simulink model "GHAME_Model_2018b"  (R2018b)
settings: Solver=ode2  StartTime=0.0  StopTime=Sim.simulation.duration  FixedStep=Sim.sample_time  RelTol=1e-3
undefined symbols (not defined in the file): Data, IC, Sim, UNC, v0_BE_B
libraries: simulink_extras x8, sharedutil x2
(part 2 of 2)

== matlab function GHAME_Model_2018b/GHAME Airframe/Forces and Moments/PROPULSION/Subsystem/Updating mass and inertia ==
  data: IBBB output size=[3 3]; IBBBdot output; fmdot input; fmasse input; vmass output size=[1 1]; Sim parameter; stop_flag output
function [IBBB, IBBBdot, vmass, stop_flag] = mass(fmdot, fmasse, Sim)
% mass
% -------------------------------------------------------------------------
% Updates the vehicle total mass, mass derivative, inertia tensor, and 
% inertia time derivative as a function of expended fuel. The mass 
% properties are interpolated between the full and empty tank conditions. 
% A stop flag is generated when the remaining fuel mass approaches zero.
%
% INPUTS:
%   fmdot   - Fuel mass flow rate (fuel consumption rate) [kg/s]
%   fmasse  - Expended fuel mass [kg]
%
% OUTPUTS:
%   vmass     - Current vehicle mass [kg]
%   vmassdot  - Time derivative of vehicle mass [kg/s]
%   IBBB      - Current inertia tensor [3x3]
%   IBBBdot   - Time derivative of inertia tensor [3x3/s]
%   stop_flag - Boolean flag (1 if fuel is exhausted, 0 otherwise)

fmass_init = Sim.vehicle.mass.fuel;
fmass_full = Sim.vehicle.mass.fuel_full;
vmass_init = Sim.vehicle.mass.current;
IBBB0  = Sim.vehicle.inertia.IBBB0;
IBBB1  = Sim.vehicle.inertia.IBBB1;

% Updating vehicle mass and fuel mass based on expended fuel
vmass = vmass_init - fmasse;       % Current vehicle mass
fmass = fmass_init - fmasse;       % Remaining fuel mass

% Time derivative of vehicle mass (negative fuel consumption rate)
vmassdot = -fmdot;

% Compute interpolation ratio (0 = full tank, 1 = empty tank)
mass_ratio = fmass / fmass_full;

% Difference in inertia between full and empty tank
dI = IBBB0 - IBBB1;

% Interpolate inertia tensor based on current fuel state
IBBB = IBBB1 + dI * mass_ratio;

% Compute inertia tensor time derivative using chain rule
IBBBdot = (-fmdot / fmass_full) * dI;

% Generate stop flag when fuel is nearly exhausted
stop_flag = (fmass <= 1e-6);

end

== matlab function GHAME_Model_2018b/GHAME Airframe/Environment/ENVIRONMENT/Wind and Turbulence/Wind Computation ==
  settings: updateMethod=CONTINUOUS
  data: Vwind input; VTAD input; VAEDS input; VAED output; Sim parameter; VAEDSD output
function [VAED, VAEDSD]  = wind(Vwind, VTAD, VAEDS, Sim)
    % Wind Computes atmospheric properties, wind, and turbulence.
    %
    % States:
    % VAED   - Wind velocity in geodetic coordinates - m/s
    % VAEDS  - Smoothed wind velocity in geodetic coord - m/s
    % VAEDSD - Smoothed wind velocity derivative - m/s

    mturb = Sim.mode.mturb;
    mwind = Sim.mode.mwind;
    
    % Constants
    twind = 10;           % Wind smoothing time constant
    if mwind > 0
        % Compute wind components in geodetic coordinates
        VAED_RAW = [Vwind(1);  % North (meridional)
                    Vwind(2);  % East  (zonal)
                    0];      % Vertical (positive up)
    
        % Smoothing wind by filtering with time constant 'twind' sec
        VAEDSD = (VAED_RAW - VAEDS) * (1 / twind);
        VAED   = VAEDS;
    else
        VAEDSD = [0; 0; 0];
        VAED   = [0; 0; 0];
    end
    
    % Add Dryden turbulence
    if mturb > 0
        VAED = VAED + VTAD;
    else 
    end

end

== matlab function GHAME_Model_2018b/GHAME Airframe/Environment/ENVIRONMENT/Gravity Calculation ==
  data: time input; SBII input; GRAVG output; IC parameter; Sim parameter
function GRAVG  = cad_grav84(time, SBII, IC, Sim)
  
    % Extract Constants
    SMAJOR_AXIS = Sim.earth.SMAJOR_AXIS;
    C20         = Sim.earth.C20;
    REARTH      = Sim.earth.REARTH;
    GW_CLONG    = Sim.earth.GW_CLONG;
    GM          = Sim.earth.GM;

    WEII3 = IC.WEII3;

    % Initialize output
    GRAVG = zeros(3,1);

    % Compute geocentric coordinates
    [lonc, latc, altc] = cad_geoc_in(SBII, time, REARTH, WEII3, GW_CLONG);

    % Compute the gravitational acceleration
    dbi = norm(SBII); % Magnitude of position vector
    dum1 = GM / (dbi^2);
    dum2 = 3 * sqrt(5);
    dum3 = (SMAJOR_AXIS / dbi)^2;

    gravg1 = -dum1 * dum2 * C20 * dum3 * sin(latc) * cos(latc);
    gravg2 = 0;
    gravg3 = dum1 * (1 + dum2 / 2 * C20 * dum3 * (3 * sin(latc)^2 - 1));

    % Assign values
    GRAVG(1) = gravg1;
    GRAVG(2) = gravg2;
    GRAVG(3) = gravg3;
end

function [lonc, latc, altc] = cad_geoc_in(SBII, time, REARTH, WEII3, GW_CLONG)

    % Extract position components
    sbii1 = SBII(1);
    sbii2 = SBII(2);
    sbii3 = SBII(3);

    % Compute geodetic latitude
    dbi = norm(SBII);
    latc = asin(sbii3 / dbi);

    % Compute altitude
    altc = dbi - REARTH;

    % Compute longitude
    dum4 = asin(sbii2 / sqrt(sbii1^2 + sbii2^2));

    % Resolving multi-valued arcsin function
    if sbii1 >= 0 && sbii2 >= 0
        lon_cel = dum4; % Quadrant I
    elseif sbii1 < 0 && sbii2 >= 0
        lon_cel = pi - dum4; % Quadrant II
    elseif sbii1 < 0 && sbii2 < 0
        lon_cel = pi - dum4; % Quadrant III
    else
        lon_cel = 2 * pi + dum4; % Quadrant IV
    end

    lonc = lon_cel - WEII3 * time - GW_CLONG;

    % Adjust longitude to be in the range (-pi, pi)
    if lonc > pi
        lonc = -(2 * pi - lonc);
    end
end

== matlab function GHAME_Model_2018b/GHAME Airframe/Forces and Moments/PROPULSION/Thrust and fuel use ==
  data: rho input; Mach input; alphax input; DVBA input; Throttle input; pdynmc input; Thrust output; fmdot output; Data parameter; Sim parameter; cx_prop output; Throttle output; pdynmc output
function [ Thrust, fmdot, cx_prop, Throttle, pdynmc] = thrust(rho, Mach, alphax, DVBA, Throttle, pdynmc, Data, Sim)
% thrust
% -------------------------------------------------------------------------
% Computes the engine thrust, fuel mass depletion rate, and propulsive
% force coefficient for the vehicle. Thrust is modeled as a function of
% Mach number, throttle setting, angle of attack, and atmospheric density.
%
% INPUTS:
%   rho          - Atmospheric density [kg/m^3]
%   Mach         - Mach number [-]
%   alphax       - Angle of attack [rad]
%   DVBA         - True airspeed (speed of vehicle wrt air) [m/s]
%   Data         - Struct with engine coefficient tables:
%                    Data.Constants.Engine.ThrustCoefficients
%   Throttle     - Throttle command input [-]
%   Sim_Extender - Scaling factor for simulation time [s]
%   pdynmc       - Dynamic pressure [Pa]
%   acowl        - Engine cowl area scaling factor [-]
%   IC           - Struct with constants (requires IC.AGRAV = gravity [m/s^2])
%   refa         - Reference area [m^2]
%
% OUTPUTS:
%   Thrust       - Propulsive thrust force [N]
%   fmdot        - Fuel mass depletion rate [kg/s]
%   cx_prop      - Propulsive force coefficient [-]
%

    % Constants
    thrtl_idle   = 0.05;   % Minimum throttle setting
    thrtl_max    = 2;      % Maximum throttle setting
    AGRAV        = Sim.earth.AGRAV;    % Gravitational acceleration [m/s^2]
    Sim_Extender = Sim.simulation.Sim_Extender;
    acowl        = Sim.vehicle.acowl;
    refa         = Sim.vehicle.geometry.refa;

    % Breakpoints from engine coefficient tables
    Mach_vec     = Data.ThrustCoefficients.Mach_vec;
    alpha_vec    = Data.ThrustCoefficients.alpha_vec;
    throttle_vec = Data.ThrustCoefficients.throttle_vec;

    % Tables for thrust modeling
    capture_area_tab = Data.ThrustCoefficients.Capture_A;
    SPI_tab          = Data.ThrustCoefficients.SPI_tab;

    % Apply throttle limits
    Throttle = max(min(Throttle, thrtl_max), thrtl_idle);

    % Interpolate Specific Impulse (SPI) from Mach-throttle table
    SPI = interp2(Mach_vec, throttle_vec, SPI_tab, Mach, Throttle, 'linear');

    % Interpolate capture area from Mach-alpha table
    capture_area = interp2(Mach_vec, alpha_vec, capture_area_tab, Mach, alphax, 'linear');

    % Compute thrust [N]
    Thrust = SPI * 0.029 * Throttle * AGRAV * rho * DVBA * capture_area * acowl;

    % Compute fuel mass depletion rate [kg/s]
    fmdot = Thrust / (SPI * AGRAV * Sim_Extender);

    % Compute propulsive force coefficient [-]
    cx_prop = Thrust / (Throttle * pdynmc * refa);

end

== matlab function GHAME_Model_2018b/GHAME Airframe/Environment/ENVIRONMENT/Atmosphere calculation ==
  data: rho output; press output; tempk output; vsound output; alt_km input
function [rho, press, tempk,vsound] = us76_nasa2002(alt_km)
    % 1976 US Standard Atmosphere Model
    % Inputs:
    %   z  - Altitude (km)
    % Outputs:
    %   d  - Density (kg/m^3)
    %   p  - Pressure (Pa)
    %   t  - Temperature (K)
    %   s  - Speed of sound (m/s)
    %   status - Returns 0 if altitude is in range, 1 if out of range

    % Initialize all outputs to avoid "not fully defined" errors
  
    rho = 0;
    press = 0;
    tempk = 0;
    vsound = 0;

    % Constants
    ro = 6356.766;  % Earth radius (km)
    go = 9.80665;   % Gravity (m/s^2)
    wmo = 28.9644;  % Molecular weight (dimensionless)
    rs = 8314.32;   % Universal gas constant (J/kmol-K)

    % Altitude table (km)
    zs = [0, 11.019, 20.063, 32.162, 47.35, 51.413, 71.802, 86, 91, 94, ...
          97, 100, 103, 106, 108, 110, 112, 115, 120, 125, 130, 135, 140, ...
          145, 150, 155, 160, 165, 170, 180, 190, 210, 230, 265, 300, 350, ...
          400, 450, 500, 550, 600, 650, 700, 750, 800, 850, 900, 950, 1000];

    % Temperature table (K)
    tms = [288.15, 216.65, 216.65, 228.65, 270.65, 270.65, 214.65, ...
           186.95, 186.87, 187.74, 190.40, 195.08, 202.23, 212.89, ...
           223.29, 240.00, 264.00, 300.00, 360.00, 417.23, 469.27, ...
           516.59, 559.63, 598.78, 634.39, 666.80, 696.29, 723.13, ...
           747.57, 790.07, 825.31, 878.84, 915.78, 955.20, 976.01, ...
           990.06, 995.83, 998.22, 999.24, 999.67, 999.85, 999.93, ...
           999.97, 999.99, 999.99, 1000, 1000, 1000, 1000];

    % Molecular weight table
    wms = [28.9644, 28.9644, 28.9644, 28.9644, 28.9644, 28.9644, ...
           28.9644, 28.9522, 28.8890, 28.7830, 28.6200, 28.3950, ...
           28.1040, 27.7650, 27.5210, 27.2680, 27.0200, 26.6800, ...
           26.2050, 25.8030, 25.4360, 25.0870, 24.7490, 24.4220, ...
           24.1030, 23.7920, 23.4880, 23.1920, 22.9020, 22.3420, ...
           21.8090, 20.8250, 19.9520, 18.6880, 17.7260, 16.7350, ...
           15.9840, 15.2470, 14.3300, 13.0920, 11.5050, 9.7180, ...
           7.9980, 6.5790, 5.5430, 4.8490, 4.4040, 4.1220, 3.9400];

    % Pressure table (hPa converted to Pa)
    ps = [1013.25, 226.32, 54.7487, 8.68014, 1.10905, 0.66938, ...
          0.039564, 3.7338e-03, 1.5381e-03, 9.0560e-04, 5.3571e-04, ...
          3.2011e-04, 1.9742e-04, 1.2454e-04, 9.3188e-05, 7.1042e-05, ...
          5.5547e-05, 4.0096e-05, 2.5382e-05, 1.7354e-05, 1.2505e-05, ...
          9.3568e-06, 7.2028e-06, 5.6691e-06, 4.5422e-06, 3.6930e-06, ...
          3.0395e-06, 2.5278e-06, 2.1210e-06, 1.5271e-06, 1.1266e-06, ...
          6.4756e-07, 3.9276e-07, 1.7874e-07, 8.7704e-08, 3.4498e-08, ...
          1.4518e-08, 6.4468e-09, 3.0236e-09, 1.5137e-09, 8.2130e-10, ...
          4.8865e-10, 3.1908e-10, 2.2599e-10, 1.7036e-10, 1.3415e-10, ...
          1.0873e-10, 8.9816e-11, 7.5138e-11] * 100;

    % Check altitude range
    if alt_km < 0 || alt_km > 1000
        rho = 0; press = 0; tempk = 0; vsound = 0;
        return;
    end

    % Find altitude index using bisection search
    i = 0;
    upper = length(zs) - 1;
    while (upper - i > 1)
        test = floor((i + upper) / 2);
        if alt_km > zs(test)
            i = test;
        else
            upper = test;
        end
    end

    if i < 7
        zl = ro * zs(i) / (ro + zs(i));
        zu = ro * zs(i+1) / (ro + zs(i+1));
        wm = wmo;
        ht = ro * alt_km / (ro + alt_km);
        g = (tms(i+1) - tms(i)) / (zu - zl);

        if g ~= 0
            press = ps(i) * (tms(i) / (tms(i) + g * (ht - zl)))^((go * wmo) / (rs * g * 0.001));
        else
            press = ps(i) * exp(-(go * wmo * (ht * 1000 - zl * 1000)) / (rs * tms(i)));
        end
        tempk = tms(i) + g * (ht - zl);
    else
        % Non-tropospheric layers
        if i == 7
            tempk = tms(8);
        elseif i >= 8 && i < 15
            tempk = 263.1905 - 76.3232 * sqrt(1 - ((alt_km - 91) / 19.9429)^2);
        elseif i >= 15 && i < 18
            tempk = 240 + 12 * (alt_km - 110);
        elseif i >= 18
            xi = (alt_km - 120) * (ro + 120) / (ro + alt_km);
            tempk = 1000 - 640 * exp(-0.01875 * xi);
        end

        % Interpolating pressure and molecular weight
        j = i;
        if i == 47, j = i - 1; end

        z0 = zs(j);
        z1 = zs(j+1);
        z2 = zs(j+2);

        wma = wms(j) * (alt_km - z1) * (alt_km - z2) / ((z0 - z1) * (z0 - z2)) + ...
              wms(j+1) * (alt_km - z0) * (alt_km - z2) / ((z1 - z0) * (z1 - z2)) + ...
              wms(j+2) * (alt_km - z0) * (alt_km - z1) / ((z2 - z0) * (z2 - z1));

        alpa = log(ps(j)) * (alt_km - z1) * (alt_km - z2) / ((z0 - z1) * (z0 - z2)) + ...
               log(ps(j+1)) * (alt_km - z0) * (alt_km - z2) / ((z1 - z0) * (z1 - z2)) + ...
               log(ps(j+2)) * (alt_km - z0) * (alt_km - z1) / ((z2 - z0) * (z2 - z1));

        alpb = alpa;
        wmb = wma;

        if i ~= 7 && i ~= 47
            j = j - 1;
            z0 = zs(j);
            z1 = zs(j+1);
            z2 = zs(j+2);
            alpb = log(ps(j)) * (alt_km - z1) * (alt_km - z2) / ((z0 - z1) * (z0 - z2)) + ...
                   log(ps(j+1)) * (alt_km - z0) * (alt_km - z2) / ((z1 - z0) * (z1 - z2)) + ...
                   log(ps(j+2)) * (alt_km - z0) * (alt_km - z1) / ((z2 - z0) * (z2 - z1));

            wmb = wms(j) * (alt_km - z1) * (alt_km - z2) / ((z0 - z1) * (z0 - z2)) + ...
                  wms(j+1) * (alt_km - z0) * (alt_km - z2) / ((z1 - z0) * (z1 - z2)) + ...
                  wms(j+2) * (alt_km - z0) * (alt_km - z1) / ((z2 - z0) * (z2 - z1));
        end

        press = 100 * exp((alpa + alpb) / 2);
        wm = (wma + wmb) / 2;
    end

    % Compute density and speed of sound
    rho = (wm * press) / (rs * tempk);
    vsound = sqrt(1.4 * press / rho);
end

== matlab function GHAME_Model_2018b/INS/INS/Inertial Navigation System ==
  settings: updateMethod=DISCRETE
  data: muc output; lonc output; latc output; psivdc output; thtvdc output; WBICB output; FSPCB output; dvbec output; SBII input; VBII input; TBI input; WBIB input; FSPB input; time input; alphacx output; betacx output; altc output; Sim parameter; nzc output; IC parameter
function [muc, lonc, latc, psivdc, thtvdc, WBICB, FSPCB, dvbec, ...
    alphacx, betacx, altc, nzc] = ins(SBII, VBII, TBI, WBIB, FSPB, ...
    time, Sim, IC)
%
% INS  Inertial Navigation System model.
%
% This function computes navigation states and derived flight quantities
% from inertial position, velocity, attitude, angular rates, and specific
% force inputs.
%
% In the current implementation, only gyro-related error sources are 
% modeled. Extensions toward a higher-fidelity INS (e.g., including
% accelerometer errors, GPS aiding, or star tracker updates) can be
% incorporated by building the corresponding subsystems and error models.
%
% Future extensions may include explicit integration schemes for:
%   RICID, EVBID, ESBID, RICI, EVBI, ESBI
% As described in Modeling and Simulation of Aerospace Vehicles, Zipfel

% Constants
SMAJOR_AXIS = Sim.earth.SMAJOR_AXIS;
FLATTENING  = Sim.earth.FLATTENING;
AGRAV       = Sim.earth.AGRAV;
DEG         = Sim.constants.DEG;
PI          = Sim.constants.PI;
EPS         = Sim.constants.EPS;
SMALL       = Sim.constants.SMALL;
RAD         = Sim.constants.RAD;

% Conditions
GW_CLONG    = Sim.earth.GW_CLONG;
WEII3       = IC.WEII3;
mnoise      = Sim.mode.mnoise;      % Activate noise
dt          = Sim.sample_time;      % Sample time

% Gyro Errors
EWALKG = 0.10*pi/180*1/60;                           % Gyro random walk intensity - rad/hr
EMISG  = [1.1e-4; 1.1e-4; 1.1e-4];                   % Gyro misalignment          - rad
ESCALG = [2.0e-5; 2.0e-5; 2.0e-5] ;                  % Gyro scale factor          - parts
EBIASG = [1.0e-6; 1.0e-6; 1.0e-6] ; % 0.2 deg/hour   % Gyro bias                  - rad/s

EUNBG  = [0; 0; 0];                                  % Gyro cluster misalignment - rad

% Acceleration Errors
%EWALKA  = [0; 0; 0];                       % Accel random bias         - m/s2
%EMISA   = [1.1e-4; 1.1e-4;1.1e-4];         % Accel misalignment        - rad
%ESCALA  = [5.0e-4; 5.0e-4; 5.0e-4];        % Accel scale factor        - parts
%EBIASA  = [3.56e-3; 3.56e-3; 3.56e-3] ;    % Accel bias                - m/s²

% Initialization case
TBIC = TBI;
FSPCB = FSPB;
WBICB = WBIB;
SBIIC = SBII;
VBIIC = VBII;

if mnoise > 0
    WBICB = ins_gyro(WBIB, FSPB, EUNBG, EMISG, ESCALG, EBIASG, EWALKG, dt);
end

% Compute the inertial velocity component due to Earth's rotation
VEIC = zeros(3,1);
VEIC(1) = -WEII3 * SBIIC(2);
VEIC(2) = WEII3 * SBIIC(1);
VEIC(3) = 0;

% Compute the velocity relative to the rotating Earth
VBEIC = VBIIC - VEIC;

% Transform to body frame
VBECB = TBIC * VBEIC;

% Compute the magnitude of the velocity vector in body frame
dvbec = norm(VBECB);

% Compute incidence angles from INS
alphac = atan2(VBECB(3), VBECB(1));
betac = asin(VBECB(2) / dvbec);

alphacx = alphac * DEG;
betacx = betac * DEG;

% Incidence angles in load factor plane (aeroballistic)
dum = VBECB(1) / dvbec;
dum = max(min(dum, 1), -1); % Clamp value between -1 and 1
alppc = acos(dum);

if abs(VBECB(2)) < EPS
    phipc = (VBECB(3) > 0) * 0 + (VBECB(3) < 0) * PI;
else
    phipc = atan2(VBECB(2), VBECB(3));
end

% Get longitude, latitude, altitude from INS
[lonc, latc, altc] = cad_geo84_in(SBIIC, time, SMAJOR_AXIS, FLATTENING, WEII3, GW_CLONG, SMALL, RAD);

% Get transformation matrix of geodetic wrt inertial coordinates
TDCI = cad_tdi84(lonc, latc, time, GW_CLONG, WEII3);

% Compute geodetic velocity from INS
VBECD = TDCI * VBEIC;

% Compute flight path angles
if VBECD(1) == 0 && VBECD(2) == 0
    psivdc = 0;
    thtvdc = 0;
else
    psivdc = atan2(VBECD(2), VBECD(1));
    thtvdc = atan2(-VBECD(3), sqrt(VBECD(1)^2 + VBECD(2)^2));
end

% Compute Euler angles from INS
TBD = TBIC * TDCI';
tbd13 = TBD(1,3);
tbd11 = TBD(1,1);
tbd33 = TBD(3,3);
tbd12 = TBD(1,2);
tbd23 = TBD(2,3);

% Pitch angle
if abs(tbd13) < 1
    thtbdc = asin(-tbd13);
    cthtbd = cos(thtbdc);
else
    thtbdc = sign(-tbd13) * PI / 2;
    cthtbd = EPS;
end

cpsi = tbd11 / cthtbd;
cpsi = max(min(cpsi, 1 - EPS), -1 + EPS);
cphi = tbd33 / cthtbd;
cphi = max(min(cphi, 1 - EPS), -1 + EPS);

% Yaw and roll angle
psibdc = acos(cpsi) * sign(tbd12);
phibdc = acos(cphi) * sign(tbd23);

num = tan(phibdc) + tan(betac) *...
    (tan(thtbdc)*cos(alphac)/cos(phibdc) - sin(alphac)/cos(thtbdc));

% Denominator term of atan2
den = 1 + tan(thtbdc)*sin(alphac)./(cos(betac).*cos(phibdc));

% Aerodynamic roll angle
muc = atan2(num, den);

% Normal load factor
nzc = -FSPCB(3)/AGRAV;

end

function WBICB = ins_gyro(WBIB, FSPB, EUNBG, EMISG, ESCALG, EBIASG, EWALKG, dt)

% Cluster misalignment + scale factor
EGB = diag(ESCALG) + skew_sym(EMISG);
EMISCG = EGB * WBIB;
EMSBG = EBIASG + EMISCG;

% Spin axis sensitivity (mass unbalance)
EUG = EUNBG .* FSPB;

% Random walk
sigma = EWALKG/(sqrt(dt));
EWG   = sigma .* randn(3,1);

% Total error
EWBIB = EMSBG + EUG + EWG;

% Measured body rate
WBICB = WBIB + EWBIB;
end

function S = skew_sym(v)
S = [  0    -v(3)  v(2);
    v(3)   0   -v(1);
    -v(2)  v(1)   0  ];
end

% function EGRAVI = ins_grav(ESBI, SBIIC, dbi, GM)
% dbic = norm(SBIIC);
% ed = dbic - dbi;
% dum = GM / dbic^3;
% EGRAVI = -dum * ESBI - 3 * dum * ed / dbic * SBIIC;
% end
% 
% function EFSPB = ins_accl(FSPB, EMISA, ESCALA, EBIASA)
% EAB = diag(ESCALA) + skew_sym(EMISA);
% EFSPB = EBIASA + EAB * FSPB;
% end

function [lon, lat, alt] = cad_geo84_in(SBII, time, SMAJOR_AXIS, FLATTENING, WEII3, GW_CLONG, SMALL, RAD)

% Initializing variables
count = 0;
lat0 = 0;
alamda = 0;

% Compute geocentric latitude
dbi = norm(SBII); % Magnitude of SBII
latg = asin(SBII(3) / dbi);
lat = latg;

% Iterating to compute geodetic latitude and altitude
while true
    lat0 = lat;
    r0 = SMAJOR_AXIS * (1 - FLATTENING * (1 - cos(2 * lat0)) / 2 + 5 * FLATTENING^2 * (1 - cos(4 * lat0)) / 16); % Equation 4-21
    alt = dbi - r0;
    dd = FLATTENING * sin(2 * lat0) * (1 - FLATTENING / 2 - alt / r0); % Equation 4-15
    lat = latg + dd;
    count = count + 1;

    % Check for convergence
    if abs(lat - lat0) < SMALL
        break;
    end

    % Prevent infinite loop
    if count > 100
        error('Geodetic latitude does not converge in cad_geo84_in().');
    end
end

% Compute longitude
sbii1 = SBII(1);
sbii2 = SBII(2);
dum4 = asin(sbii2 / sqrt(sbii1^2 + sbii2^2));

% Resolving multi-valued arcsin function (handling quadrants)
if (sbii1 >= 0.0) && (sbii2 >= 0.0)
    alamda = dum4; % Quadrant I
elseif (sbii1 < 0.0) && (sbii2 >= 0.0)
    alamda = (180 * RAD) - dum4; % Quadrant II
elseif (sbii1 < 0.0) && (sbii2 < 0.0)
    alamda = (180 * RAD) - dum4; % Quadrant III
elseif (sbii1 > 0.0) && (sbii2 < 0.0)
    alamda = (360 * RAD) + dum4; % Quadrant IV
end

lon = alamda - WEII3 * time - GW_CLONG;

% Adjust longitude to keep within (-180, 180) degrees
if lon > (180 * RAD)
    lon = -((360 * RAD) - lon);
end
end

function TDI = cad_tdi84(lon, lat, time, GW_CLONG, WEII3)

% Compute celestial longitude of the vehicle at simulation 'time'
lon_cel = GW_CLONG + WEII3 * time + lon;

% Compute transformation matrix elements
tdi13 = cos(lat);
tdi33 = -sin(lat);
tdi22 = cos(lon_cel);
tdi21 = -sin(lon_cel);

% Construct the transformation matrix
TDI = [ tdi33 * tdi22, -tdi33 * tdi21, tdi13;
    tdi21,         tdi22,          0;
    -tdi13 * tdi22,  tdi13 * tdi21, tdi33 ];
end

== matlab function GHAME_Model_2018b/GHAME Airframe/Dynamics/NEWTON/Geodetic position update/Geodetic Position ==
  data: lon output; lon_cel output; time input; SBII input; IC parameter; lat output; alt output; Sim parameter
function [lon, lon_cel, lat, alt] = cad_geo84_in_cont(time, SBII, IC, Sim)
% cad_geo84_in_cont
% -------------------------------------------------------------------------
% Converts the inertial position vector [s_BI]^I into geodetic coordinates:
% geodetic longitude, latitude, and altitude above the reference ellipsoid.
%
% INPUTS:
%   time   - Current simulation time [s]
%   SBII   - 3x1 position vector of the body in inertial coordinates [m]
%   IC     - Struct containing ellipsoid parameters:
%               FLATTENING   = flattening factor f [-]
%               SMAJOR_AXIS  = semi-major axis a [m]
%               GW_CLONG     = Greenwich longitude at initial epoch [rad]
%   WEII3  - Earth rotation rate about inertial Z-axis [rad/s]
%
% OUTPUTS:
%   lon    - Geodetic longitude [rad]
%   lat    - Geodetic latitude [rad]
%   alt    - Geometric altitude above the ellipsoid [m]
%
% METHOD:
%   1. Extract Cartesian inertial position (x, y, z).
%   2. Compute inertial longitude and convert it to geodetic longitude
%      by subtracting Earth rotation and Greenwich reference.
%   3. Normalize longitude to the range (-π, π).
%   4. Estimate geocentric latitude, then apply correction for ellipsoidal
%      Earth to obtain geodetic latitude.
%   5. Compute altitude using the radius of curvature in the prime vertical.
%
% -------------------------------------------------------------------------

    % Extract constants from Sim
    FLATTENING  = Sim.earth.FLATTENING;
    SMAJOR_AXIS = Sim.earth.SMAJOR_AXIS;
    GW_CLONG    = Sim.earth.GW_CLONG;
    
    WEII3 = IC.WEII3;

    % Earth's eccentricity squared
    e2 = 2 * FLATTENING - FLATTENING^2;

    % Extract position in inertial coordinates
    x = SBII(1);
    y = SBII(2);
    z = SBII(3);

    % Compute longitude from inertial position
    lon_inertial = atan2(y, x);
    lon = lon_inertial - WEII3 * time - GW_CLONG;

    % Normalize longitude to (-pi, pi)
    lon = atan2(sin(lon), cos(lon));

    % Compute celestial longitude of the vehicle at simulation 'time'
    lon_cel = GW_CLONG + WEII3 * time + lon;

    % Compute intermediate quantities
    rho = sqrt(x^2 + y^2);              % projection in equatorial plane
    dbi = sqrt(x^2 + y^2 + z^2);        % distance from Earth's center

    % Geocentric latitude
    lat_gc = atan2(z, rho);

    % Geodetic latitude (iterative correction replaced by closed form approx.)
    lat = atan2(z + e2 * SMAJOR_AXIS * sin(lat_gc)^3, ...
                rho - e2 * SMAJOR_AXIS * cos(lat_gc)^3);

    % Radius of curvature in the prime vertical
    N = SMAJOR_AXIS / sqrt(1 - e2 * sin(lat)^2);

    % Altitude above ellipsoid
    alt = rho / cos(lat) - N;
end

== matlab function GHAME_Model_2018b/GHAME Airframe/Dynamics/NEWTON/Geodetic position update/TM Inertial to Geocentric ==
  data: TDI input; lat input; alt input; TGI output; TDI output; lat output; Sim parameter; alt output
function [TGI, TDI, lat, alt] = cad_tgi84(TDI, lat, alt, Sim)
% cad_tgi84
% -------------------------------------------------------------------------
% Computes the transformation matrix [T]^{GI}, which transforms vectors
% from the inertial coordinate system (I) to the geocentric coordinate
% system (G). The computation is based on an ellipsoidal Earth model using
% the first and second flattening terms (f, f^2).
%
% INPUTS:
%   TDI  - 3x3 transformation matrix [T]^{DI} (Inertial -> Geodetic)
%   lat  - Geodetic latitude [rad]
%   alt  - Geometric altitude above the ellipsoid [m]
%   IC   - Struct containing ellipsoid parameters:
%              FLATTENING   = flattening factor f [-]
%              SMAJOR_AXIS  = semi-major axis a [m]
%
% OUTPUT:
%   TGI  - 3x3 transformation matrix [T]^{GI} (Inertial -> Geocentric)
%

    % Extract constants from IC
    FLATTENING   = Sim.earth.FLATTENING;    % ellipsoid flattening f [-]
    SMAJOR_AXIS  = Sim.earth.SMAJOR_AXIS;   % semi-major axis a [m]
    
    % Compute Earth's radius to ellipsoid surface (r0)
    r0 = SMAJOR_AXIS * (1 - FLATTENING * (1 - cos(2 * lat)) / 2 + ...
        5 * FLATTENING^2 * (1 - cos(4 * lat)) / 16); 
    
    % Compute normal deflection angle (dd)
    dd = FLATTENING * sin(2 * lat) * (1 - FLATTENING / 2 - alt / r0); 
    
    % Transformation matrix of Geocentric wrt Geodetic coordinates [T]^{GD}
    TGD = [cos(dd), 0, -sin(dd);
           0,       1,  0;
           sin(dd), 0,  cos(dd)];
    
    % Compute transformation matrix of Geocentric wrt Inertial coordinates
    TGI = TGD * TDI;

end

== matlab function GHAME_Model_2018b/GHAME Airframe/Dynamics/NEWTON/Geodetic position update/TM Inertial to Geodetic ==
  data: lon_cel input; TDI output; lat input; lat output
function [TDI, lat] = cad_tdi84(lon_cel, lat)
% cad_tdi84
% -------------------------------------------------------------------------
% Computes the transformation matrix [T]^{DI}, which transforms vectors
% from the inertial coordinate system (I) to the geodetic coordinate system (D).
%
% INPUTS:
%   time   - Current simulation time [s]
%   lon    - Geodetic longitude of the vehicle [rad]
%   lat    - Geodetic latitude of the vehicle [rad]
%   WEII3  - Earth rotation rate about inertial Z-axis [rad/s]
%   IC     - Struct containing initial conditions
%              IC.GW_CLONG = Greenwich longitude at initial epoch [rad]
%
% OUTPUT:
%   TDI    - 3x3 transformation matrix [T]^{DI}
%
% METHOD:
%   1. Compute the celestial longitude of the vehicle as a function of
%      Greenwich longitude, Earth rotation, simulation time, and geodetic longitude.
%   2. Form intermediate trigonometric terms.
%   3. Assemble the direction cosine matrix [T]^{DI}.
%
% -------------------------------------------------------------------------

    %GW_CLONG = IC.GW_CLONG;

    % Compute celestial longitude of the vehicle at simulation 'time'
    %lon_cel = GW_CLONG + WEII3 * time + lon;

    % Compute transformation matrix elements
    tdi13 = cos(lat);
    tdi33 = -sin(lat);
    tdi22 = cos(lon_cel);
    tdi21 = -sin(lon_cel);

    % Construct the transformation matrix
    TDI = [ tdi33 * tdi22, -tdi33 * tdi21, tdi13;
            tdi21,         tdi22,          0;
           -tdi13 * tdi22,  tdi13 * tdi21, tdi33 ];
end

== matlab function GHAME_Model_2018b/GHAME Airframe/Forces and Moments/FORCE/Aerodynamic moments ==
  data: c_moment input; pdynmc input; FMB output; Sim parameter
function FMB = computeMoment(c_moment, pdynmc, Sim)
% computeMoment
% -------------------------------------------------------------------------
% Computes the aerodynamic moment vector in the body coordinate system.
% The aerodynamic moments are obtained from the non-dimensional moment
% coefficients, scaled by dynamic pressure, reference area, and reference
% lengths.
%
% INPUTS:
%   pdynmc  - Dynamic pressure [Pa]
%   cll     - Non-dimensional rolling moment coefficient [-]
%   clm     - Non-dimensional pitching moment coefficient [-]
%   cln     - Non-dimensional yawing moment coefficient [-]

    refa = Sim.vehicle.geometry.refa;
    refb = Sim.vehicle.geometry.refb;
    refc = Sim.vehicle.geometry.refc;

    cll = c_moment(1);
    clm = c_moment(2);
    cln = c_moment(3);
%
% OUTPUT:
%   FMB     - 3x1 vector of aerodynamic moments in the body coordinate system [N·m]
%             FMB = [M_x; M_y; M_z]

    FMB = [pdynmc * refa * refb * cll;   % Rolling moment about body x-axis
           pdynmc * refa * refc * clm;   % Pitching moment about body y-axis
           pdynmc * refa * refb * cln];  % Yawing moment about body z-axis
end

== matlab function GHAME_Model_2018b/GHAME Airframe/Kinematics/KINEMATICS/skew_sym ==
  data: WBIB input; WBIB_ss output
function WBIB_ss = vec2skew(WBIB)
% Computes the 3×3 skew symmetric matrix associated with a 3×1 vector.
% The resulting matrix represents the cross product operation in matrix form.

    x = WBIB;
    
    WBIB_ss = [   0    -x(3)   x(2) ;
                x(3)     0    -x(1) ;
               -x(2)    x(1)     0   ];

end

== matlab function GHAME_Model_2018b/GHAME Airframe/Kinematics/KINEMATICS/	Orthonormalizing TBI  ==
  data: TBI input; TBI output; ortho_error output
function [TBI, ortho_error] = normalizeT(TBI)
% Enforces orthonormality of a 3×3 transformation matrix

    % Define identity matrix
    UNIT = eye(3);

    % Compute the orthonormalization correction matrix
    EE = UNIT - TBI * TBI';

    % Apply correction to TBI
    TBI = TBI + EE * TBI * 0.5;

    % Extract diagonal elements of EE
    e1 = EE(1,1);
    e2 = EE(2,2);
    e3 = EE(3,3);

    % Compute orthogonality error
    ortho_error = sqrt(e1^2 + e2^2 + e3^2);
end

== matlab function GHAME_Model_2018b/GHAME Airframe/Kinematics/KINEMATICS/Building TDI ==
  data: lon input; TDI output; lat input; time input; Sim parameter
function TDI = cad_tdi84(lon, lat, time, Sim)
% Computes the transformation matrix from the inertial coordinate system
% to the geodetic coordinate system at a given longitude, latitude, and time
% using the WGS 84 reference ellipsoid.
%
% Return output
%			      TDI(3x3) = T.M.of geodetic wrt inertial coord - ND
% Parameter input
%			      lon = geodetic longitude - rad
%                 lat = geodetic latitude - rad
%                 alt = altitude above ellipsoid - m
%
    GW_CLONG = Sim.earth.GW_CLONG;
    WEII3    = Sim.earth.WEII3;

    % Compute celestial longitude of the vehicle at simulation 'time'
    lon_cel = GW_CLONG + WEII3 * time + lon;

    % Compute transformation matrix elements
    tdi13 = cos(lat);
    tdi33 = -sin(lat);
    tdi22 = cos(lon_cel);
    tdi21 = -sin(lon_cel);

    % Construct the transformation matrix
    TDI = [ tdi33 * tdi22, -tdi33 * tdi21, tdi13;
            tdi21,         tdi22,          0;
           -tdi13 * tdi22,  tdi13 * tdi21, tdi33 ];
    
end

== matlab function GHAME_Model_2018b/GHAME Airframe/Kinematics/KINEMATICS/Euler angles ==
  data: TBD input; psibdx output; thtbdx output; phibdx output; Sim parameter
function [psibdx, thtbdx, phibdx] = euler(TBD, Sim)
% Computes the yaw, pitch, and roll Euler angles from a geodetic-to-body 
% transformation matrix.

    EPS = Sim.constants.EPS;
    DEG = Sim.constants.DEG;
    PI  = Sim.constants.PI;
 
    % Extract elements from the TBD matrix
    tbd13 = TBD(1,3);
    tbd11 = TBD(1,1);
    tbd33 = TBD(3,3);
    tbd12 = TBD(1,2);
    tbd23 = TBD(2,3);

    % Compute thtbd
    if abs(tbd13) < 1
        thtbd = asin(-tbd13);
        cthtbd = cos(thtbd);
    else
        thtbd = (PI / 2) * sign(-tbd13);
        cthtbd = EPS;
    end

    % Compute cpsi and cphi safely
    cpsi = tbd11 / cthtbd;
    if abs(cpsi) > 1
        cpsi = sign(cpsi);
    end

    cphi = tbd33 / cthtbd;
    if abs(cphi) > 1
        cphi = sign(cphi);
    end

    % Compute angles
    psibd = acos(cpsi) * sign(tbd12);
    phibd = acos(cphi) * sign(tbd23);

    % Convert to degrees
    psibdx = DEG * psibd;
    thtbdx = DEG * thtbd;
    phibdx = DEG * phibd;
    
end

== matlab function GHAME_Model_2018b/GHAME Airframe/Kinematics/KINEMATICS/Aero angles ==
  data: VBAB input; alphax output; betax output; alppx output; phipx output; Sim parameter
function [alphax, betax, alppx, phipx] = angles_vbab(VBAB, Sim)
% Computes aerodynamic angles from the air-relative velocity vector.
    
    EPS = Sim.constants.EPS;
    DEG = Sim.constants.DEG;
    PI  = Sim.constants.PI;

    % Extract velocity components
    vbab1 = VBAB(1);
    vbab2 = VBAB(2);
    vbab3 = VBAB(3);
    
    dvba = norm(VBAB);  % airspeed magnitude

    % Compute angle of attack (alpha) and sideslip angle (beta)
    alpha = atan2(vbab3, vbab1);
    beta = asin(vbab2 / dvba);

    % Convert to degrees
    alphax = alpha * DEG;
    betax = beta * DEG;

    % Compute total angle of attack (alpp)
    dum = vbab1 / dvba;
    if abs(dum) > 1
        dum = sign(dum);  % limit domain of acos
    end
    alpp = acos(dum);

    % Compute aerodynamic roll angle (phip)
    if vbab2 == 0 && vbab3 == 0
        phip = 0;
    elseif abs(vbab2) < EPS
        phip = PI * (vbab3 < 0);
    else
        phip = atan2(vbab2, vbab3);
    end

    % Convert to degrees
    alppx = alpp * DEG;
    phipx = phip * DEG;
end
